simulink model "motorModel"  (R2021b)
settings: Solver=VariableStepAuto  StartTime=0.0  StopTime=10.0  RelTol=1e-3
InitFcn:
  | V = 12
  | Ra = 7.2
  | La =0.0917
  | Kt = 0.1236
  | Kb =0.1236
  | B = 0.0004
  | J = 0.0007046
  | TL = 0
  | N1 = 1
  | N2 = 1
  | 
settings Model: Creator=keroa  LastModifiedBy=keroa

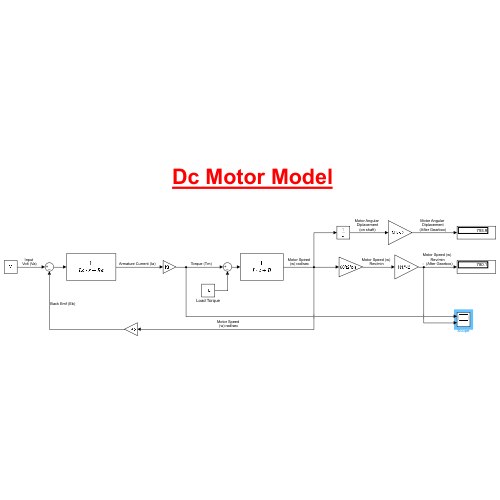
[thumbnail: Simulink's stored preview of the top-level diagram]
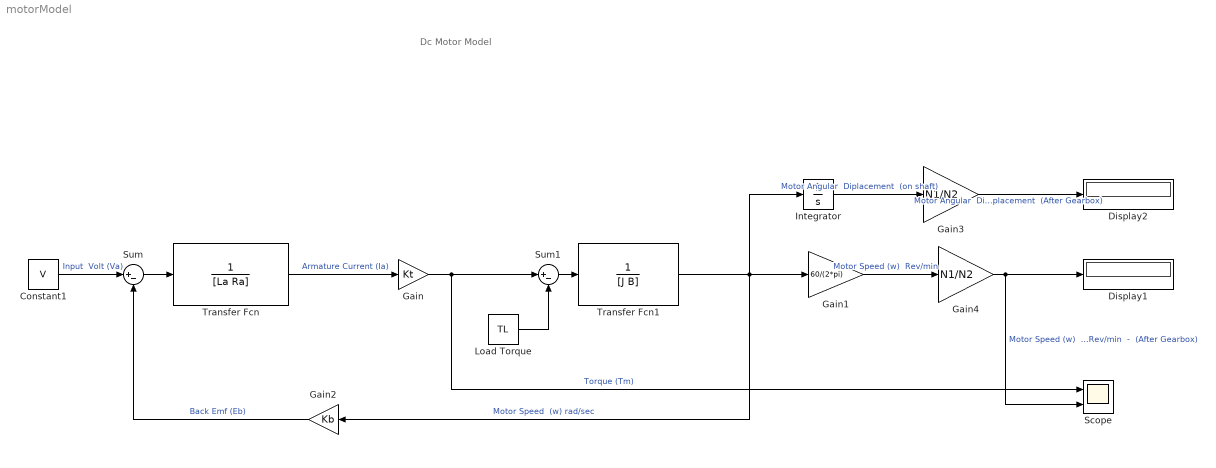
== system motorModel ==
  note: Dc Motor Model
  Constant1 : Constant  Value=V
  Display1 : Display
  Display2 : Display
  Gain : Gain  Gain=Kt
  Gain1 : Gain  Gain=60/(2*pi)
  Gain2 : Gain  Gain=Kb
  Gain3 : Gain  Gain=N1/N2
  Gain4 : Gain  Gain=N1/N2
  Integrator : Integrator
  Load Torque : Constant  Value=TL
  Scope : Scope  NumInputPorts=2
  Sum : Sum  Inputs=|+-
  Sum1 : Sum  Inputs=|+-
  Transfer Fcn : TransferFcn  Denominator=[La Ra]
  Transfer Fcn1 : TransferFcn  Denominator=[J B]
  wires:
  Constant1/1 -> Sum/1  "Input  Volt (Va)"
  Sum/1 -> Transfer Fcn/1
  Transfer Fcn/1 -> Gain/1  "Armature Current (Ia)"
  Gain/1 -> Scope/1, Sum1/1  "Torque (Tm)"
  Load Torque/1 -> Sum1/2
  Sum1/1 -> Transfer Fcn1/1
  Transfer Fcn1/1 -> Gain2/1, Gain1/1, Integrator/1  "Motor Speed  (w) rad/sec"
  Gain1/1 -> Gain4/1  "Motor Speed (w)  Rev/min"
  Integrator/1 -> Gain3/1  "Motor Angular  Diplacement  (on shaft)"
  Gain2/1 -> Sum/2  "Back Emf (Eb)"
  Gain3/1 -> Display2/1  "Motor Angular  Diplacement  (After Gearbox)"
  Gain4/1 -> Scope/2, Display1/1  "Motor Speed (w)  Rev/min  -  (After Gearbox)"
